simulink model "Robot_control_pb2"  (R2017b)
settings: Solver=ode45  StartTime=0.0  StopTime=10  RelTol=1e-3
libraries: mblibv1 x4, vrlib x1
settings Model: Creator=zigg  LastModifiedBy=alinvoicu26
settings DataIOCC: SaveFormat=StructureWithTime
settings OptimizationCC: LifeSpan=inf
settings DebuggingCC: FcnCallInpInsideContextMsg=warning  SFExecutionAtInitializationDiag=none
settings HardwareCC: ProdBitPerSizeT=32  ProdBitPerPtrDiffT=32  ProdWordSize=32  ProdHWDeviceType=Specified
settings CodeAppCC: StateflowObjectComments=on

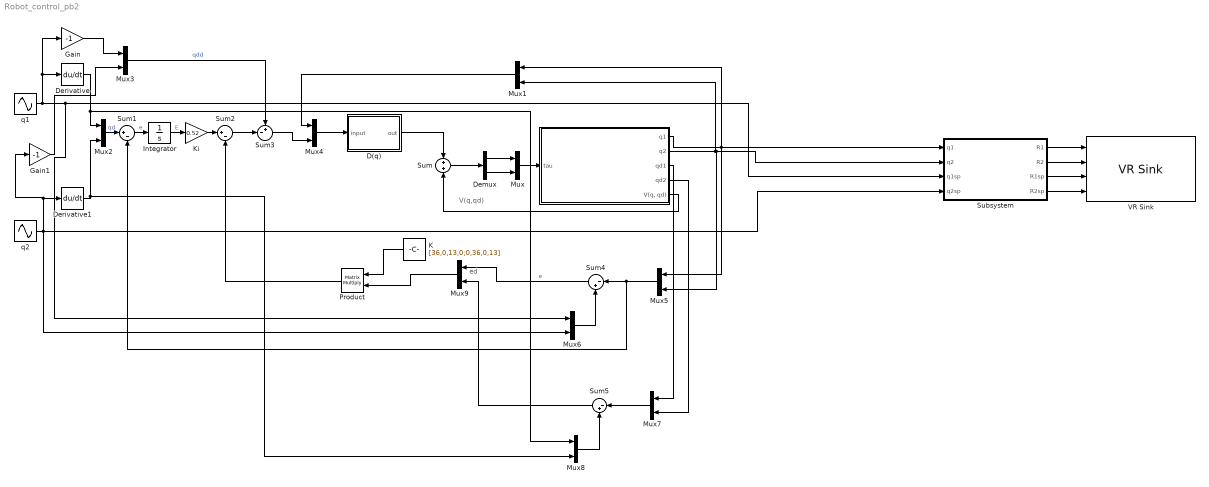
== system Robot_control_pb2 ==
  note: ed
  note: V(q,qd)
  " " : Subsystem
  D(q) : MATLAB Function  TreatAsAtomicUnit=on
  Demux : Demux  Outputs=2
  Derivative : Derivative  CoefficientInTFapproximation=100
  Derivative1 : Derivative  CoefficientInTFapproximation=100
  Gain : Gain  Gain=-1
  Gain1 : Gain  Gain=-1
  Integrator : Integrator
  K : Constant  Value=[36,0,13,0;0,36,0,13]
  Ki : Gain  Gain=0.52
  Mux{,1..9} (10 alike) : Mux  Inputs=2
  Product : Product  Multiplication=Matrix(*)
  Subsystem : Subsystem
  Sum : Sum
  Sum1 : Sum  Inputs=|+-
  Sum2 : Sum  Inputs=|+-
  Sum3 : Sum  Inputs=+-|
  Sum4 : Sum  Inputs=|-+
  Sum5 : Sum  Inputs=|-+
  VR Sink : vrlib/VR Sink  InstantiateOnLoad=on  SampleTime=0.1  ViewEnable=on  RemoteChange=off  RemoteView=off  FieldsWritten=Joint1.rotation.4.1.1.double#Joint2.rotation.4.1.1.double#Joint1_SP.rotation.4.1.1.double#Joint2_SP.rotation.4.1.1.double  WorldFileName=my_robot.wrl  AutoView=off  VideoDimensions=[]  AllowVariableSize=off  FigureProperties="{'Position', 'Name', 'Viewpoint', 'CameraBound', 'CameraDirection', 'CameraPosition', 'CameraUpVector', 'ZoomFactor', 'Antialiasing', 'Headlight', 'Lighting', 'NavPanel', 'Sound', 'StatusBar', 'Stereo3D', 'Stereo3DCameraOffset', 'Stereo3DHIT', 'ToolBar', 'Textures', 'Transparency', 'Triad', 'Wireframe', 'NavZones', 'NavMode', 'NavSpeed', 'CaptureFileFormat', 'CaptureFileName', 'Record2DCompressMethod', 'Record2DCompressQuality', 'Record2D', 'Record2DFileName', 'Record2DFPS'; [2.0000000000000000e+00   8.4000000000000000e+01   9.5800000000000000e+02   9.0400000000000000e+02], '', '', 'on', [3.1410759078128327e-02   0.0000000000000000e+00  -9.9950656036573204e-01], [-2.2544204540206194e+00   0.0000000000000000e+00   5.3842362600011839e+01], [0.0000000000000000e+00   1.0000000000000000e+00   0.0000000000000000e+00], [1.0000000000000000e+00], 'on', 'on', 'on', 'halfbar', 'on', 'on', 'off', [1.0000000149011612e-01], [0.0000000000000000e+00], 'on', 'on', 'on', 'none', 'off', 'off', 'fly', 'normal', 'tif', '%f_anim_%n.tif', 'auto', [7.5000000000000000e+01], 'off', '%f_anim_%n.avi', 'auto'}"
      settings: SourceProductBaseCode=VR
  q1 : Sin  Frequency=0.75  SampleTime=0
  q2 : Sin  Frequency=0.5  SampleTime=0
  wires:
  Subsystem/1(R1) -> VR Sink/1
  Subsystem/2(R2) -> VR Sink/2
  Subsystem/3(R1sp) -> VR Sink/3
  Subsystem/4(R2sp) -> VR Sink/4
  " "/1(q1) -> Mux5/1, Mux1/1, Subsystem/1(q1)
  " "/2(q2) -> Mux1/2, Mux5/2, Subsystem/2(q2)
  q2/1 -> Mux6/2, Gain1/1, Derivative1/1, Subsystem/4(q2sp)
  Mux/1 -> " "/1(tau)
  " "/5("V(q, qd)") -> Sum/2
  q1/1 -> Mux6/1, Subsystem/3(q1sp), Gain/1, Derivative/1
  Derivative1/1 -> Mux8/2, Mux2/2
  Derivative/1 -> Mux8/1, Mux2/1
  Mux2/1 -> Sum1/1  "qd"
  Sum1/1 -> Integrator/1  "e"
  Integrator/1 -> Ki/1  "E"
  Ki/1 -> Sum2/1
  Sum2/1 -> Sum3/2
  Gain1/1 -> Mux3/2
  Gain/1 -> Mux3/1
  Mux3/1 -> Sum3/1  "qdd"
  Mux4/1 -> D(q)/1(input)
  Mux1/1 -> Mux4/1
  Sum3/1 -> Mux4/2
  D(q)/1(out) -> Sum/1
  Sum/1 -> Demux/1
  Demux/1 -> Mux/1
  Demux/2 -> Mux/2
  Mux6/1 -> Sum4/2
  Mux8/1 -> Sum5/2
  Mux7/1 -> Sum5/1
  " "/3("qd1 ") -> Mux7/1
  " "/4("qd2 ") -> Mux7/2
  Sum4/1 -> Mux9/1  "e"
  Sum5/1 -> Mux9/2
  Product/1 -> Sum2/2
  Mux5/1 -> Sum1/2, Sum4/1
  Mux9/1 -> Product/2
  K/1 -> Product/1

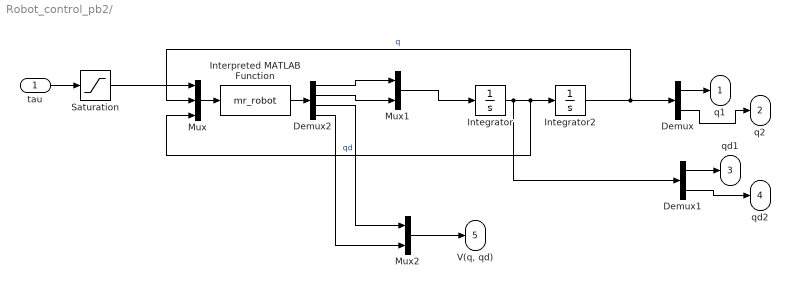
== system Robot_control_pb2/  ==
  tau : Inport
  Demux : Demux  Outputs=2
  Demux1 : Demux  Outputs=2
  Demux2 : Demux
  Integrator : Integrator
  Integrator2 : Integrator  InitialCondition=pi/2*0
  Interpreted MATLAB Function : MATLABFcn  MATLABFcn=mr_robot  OutputDimensions=4
  Mux : Mux  Inputs=3
  Mux1 : Mux  Inputs=2
  Mux2 : Mux  Inputs=2
  Saturation : Saturate  UpperLimit=1.18  LowerLimit=-1.18
  q1 : Outport
  q2 : Outport  Port=2
  "qd1 " : Outport  Port=3
  "qd2 " : Outport  Port=4
  "V(q, qd)" : Outport  Port=5
  wires:
  Integrator2/1 -> Demux/1, Mux/2  "q"
  Integrator/1 -> Demux1/1, Mux/3, Integrator2/1  "qd"
  tau/1 -> Saturation/1
  Mux/1 -> Interpreted MATLAB Function/1
  Demux/1 -> q1/1
  Demux/2 -> q2/1
  Saturation/1 -> Mux/1
  Demux1/1 -> "qd1 "/1
  Demux1/2 -> "qd2 "/1
  Interpreted MATLAB Function/1 -> Demux2/1
  Demux2/1 -> Mux1/1
  Demux2/2 -> Mux1/2
  Mux1/1 -> Integrator/1
  Demux2/3 -> Mux2/1
  Demux2/4 -> Mux2/2
  Mux2/1 -> "V(q, qd)"/1

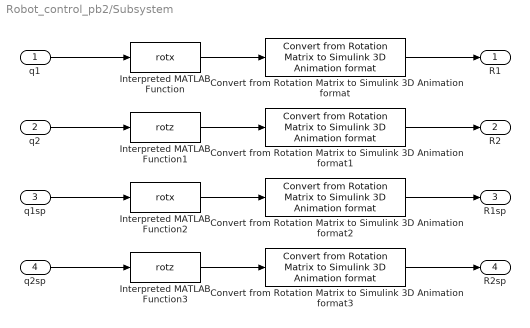
== system Robot_control_pb2/Subsystem ==
  q1 : Inport
  q2 : Inport  Port=2
  q1sp : Inport  Port=3
  q2sp : Inport  Port=4
  Convert from Rotation Matrix to Simulink 3D Animation format{,1..3} (4 alike) : mblibv1/Utilities/Convert from Rotation Matrix to Simulink 3D Animation format
      settings: SourceProductName=Simscape Multibody  SourceProductBaseCode=MS
  Interpreted MATLAB Function : MATLABFcn  MATLABFcn=rotx
  Interpreted MATLAB Function1 : MATLABFcn  MATLABFcn=rotz
  Interpreted MATLAB Function2 : MATLABFcn  MATLABFcn=rotx
  Interpreted MATLAB Function3 : MATLABFcn  MATLABFcn=rotz
  R1 : Outport
  R2 : Outport  Port=2
  R1sp : Outport  Port=3
  R2sp : Outport  Port=4
  wires:
  Convert from Rotation Matrix to Simulink 3D Animation format/1 -> R1/1
  Interpreted MATLAB Function/1 -> Convert from Rotation Matrix to Simulink 3D Animation format/1
  Interpreted MATLAB Function1/1 -> Convert from Rotation Matrix to Simulink 3D Animation format1/1
  Interpreted MATLAB Function2/1 -> Convert from Rotation Matrix to Simulink 3D Animation format2/1
  Interpreted MATLAB Function3/1 -> Convert from Rotation Matrix to Simulink 3D Animation format3/1
  q1/1 -> Interpreted MATLAB Function/1
  q2/1 -> Interpreted MATLAB Function1/1
  q1sp/1 -> Interpreted MATLAB Function2/1
  q2sp/1 -> Interpreted MATLAB Function3/1
  Convert from Rotation Matrix to Simulink 3D Animation format1/1 -> R2/1
  Convert from Rotation Matrix to Simulink 3D Animation format2/1 -> R1sp/1
  Convert from Rotation Matrix to Simulink 3D Animation format3/1 -> R2sp/1

== matlab function Robot_control_pb2/D(q) ==
  data: input input; out output
function out = fcn(input)

    q1 = input(1);
    q2 = input(2);
    A = input(3:4);
    
    out = [0.003515*cos(q2) + 0.000925*cos(q2)^2 + 0.026254, 0;
         0, 0.023625]*A;

end
